simulink model "Proj_10"  (R2017a)
settings: Solver=ode4  StartTime=0.0  StopTime=1000  FixedStep=1  RelTol=1e-3  EnableMultiTasking=on
undefined symbols (not defined in the file or in its folder): ess, mc
libraries: simulink x1
settings Model: Creator=chok1124  LastModifiedBy=Jinesh
settings OptimizationCC: LifeSpan=inf
settings DebuggingCC: SFUnexpectedBacktrackingDiag=warning  SFNoUnconditionalDefaultTransitionDiag=warning  SFExecutionAtInitializationDiag=none
settings GRTTargetCC: TargetLangStandard=C89/C90 (ANSI)  GeneratePreprocessorConditionals=Disable all
settings ConfigComp: CovMetricSettings=dw  CovHtmlReporting=on  CovSaveCumulativeToWorkspaceVar=on  CovSaveSingleToWorkspaceVar=on  CovExternalEMLEnable=off

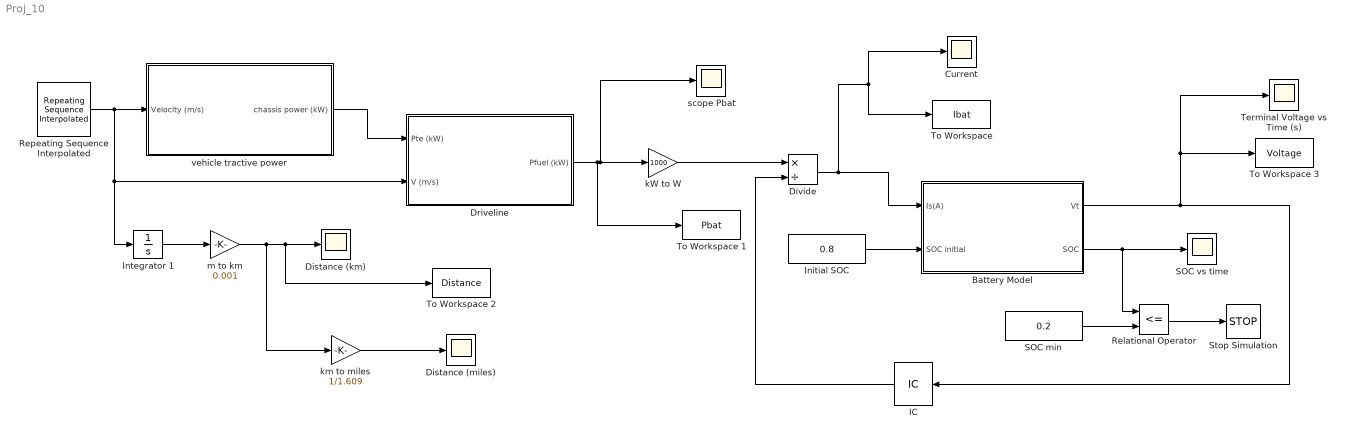
== system Proj_10 ==
  Battery Model : Subsystem
  Current : Scope
  Distance (km) : Scope
  Distance (miles) : Scope
  Divide : Product  Inputs=*/
  Driveline : Subsystem
  IC : InitialCondition  Value=345
  Initial SOC : Constant  Value=0.8
  Integrator 1 : Integrator
  Relational Operator : RelationalOperator  Operator=<=  OutDataTypeStr=boolean  RndMeth=Nearest
  Repeating Sequence Interpolated : simulink/Sources/Repeating Sequence Interpolated  OutValues=V  TimeValues=t  LookUpMeth=Interpolation-Use End Values  tsamp=1  OutMin=[]  OutMax=[]  OutDataTypeStr=double  OutputDataTypeScalingMode=double  OutDataType=fixdt(0,8)  OutScaling=2^-10
  SOC min : Constant  Value=0.2
  SOC vs time : Scope
  Stop Simulation : Stop
  Terminal Voltage vs Time (s) : Scope
  To Workspace : ToWorkspace  VariableName=Ibat  SaveFormat=Timeseries  SampleTime=-1
  To Workspace 1 : ToWorkspace  VariableName=Pbat  SaveFormat=Timeseries  SampleTime=-1
  To Workspace 2 : ToWorkspace  VariableName=Distance  SaveFormat=Timeseries  SampleTime=-1
  To Workspace 3 : ToWorkspace  VariableName=Voltage  SaveFormat=Timeseries  SampleTime=-1
  kW to W : Gain  Gain=1000
  km to miles : Gain  Gain=1/1.609
  m to km : Gain  Gain=0.001
  scope Pbat : Scope
  vehicle tractive power : Subsystem
  wires:
  Divide/1 -> Battery Model/1(Is(A)), To Workspace/1, Current/1
  Initial SOC/1 -> Battery Model/2(SOC initial)
  Battery Model/1(Vt) -> To Workspace 3/1, Terminal Voltage vs Time (s)/1, IC/1
  Battery Model/2(SOC) -> Relational Operator/1, SOC vs time/1
  SOC min/1 -> Relational Operator/2
  Relational Operator/1 -> Stop Simulation/1
  Repeating Sequence Interpolated/1 -> vehicle tractive power/1(Velocity (m/s)), Integrator 1/1, Driveline/2(V (m/s))
  Integrator 1/1 -> m to km/1
  m to km/1 -> Distance (km)/1, To Workspace 2/1, km to miles/1
  vehicle tractive power/1(chassis power (kW)) -> Driveline/1(Pte (kW))
  Driveline/1(Pfuel (kW)) -> kW to W/1, scope Pbat/1, To Workspace 1/1
  km to miles/1 -> Distance (miles)/1
  kW to W/1 -> Divide/1
  IC/1 -> Divide/2

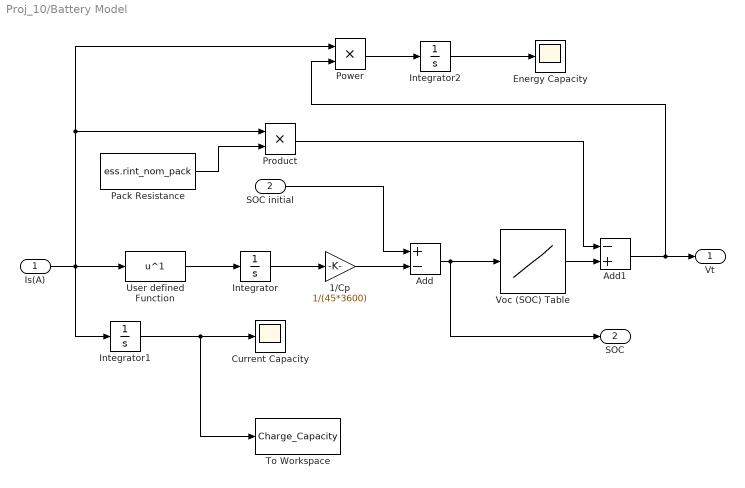
== system Proj_10/Battery Model ==
  Is(A) : Inport
  SOC initial : Inport  Port=2
  1/Cp : Gain  Gain=1/(45*3600)
  Add : Sum  Inputs=+-
  Add1 : Sum  Inputs=-+
  Current Capacity : Scope
  Energy Capacity : Scope
  Integrator : Integrator
  Integrator1 : Integrator
  Integrator2 : Integrator
  Pack Resistance : Constant  Value=ess.rint_nom_pack
  Power : Product
  Product : Product
  To Workspace : ToWorkspace  VariableName=Charge_Capacity  SaveFormat=Timeseries  SampleTime=-1
  User defined Function : Fcn  Expr=u^1
  Voc (SOC) Table : Lookup_n-D  NumberOfTableDimensions=1  BreakpointsForDimension1=ess.soc_index  Table=ess.voc_map_pack  InternalRulePriority=Speed  RndMeth=Simplest  InputSameDT=on
  Vt : Outport
  SOC : Outport  Port=2
  wires:
  Integrator/1 -> 1/Cp/1
  Is(A)/1 -> Integrator1/1, User defined Function/1, Power/1, Product/1
  User defined Function/1 -> Integrator/1
  1/Cp/1 -> Add/2
  SOC initial/1 -> Add/1
  Pack Resistance/1 -> Product/2
  Product/1 -> Add1/1
  Add/1 -> SOC/1, Voc (SOC) Table/1
  Add1/1 -> Power/2, Vt/1
  Voc (SOC) Table/1 -> Add1/2
  Integrator1/1 -> To Workspace/1, Current Capacity/1
  Power/1 -> Integrator2/1
  Integrator2/1 -> Energy Capacity/1

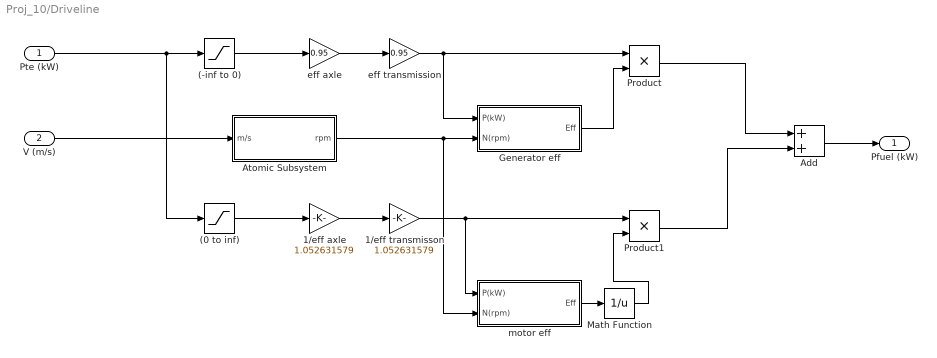
== system Proj_10/Driveline ==
  Pte (kW) : Inport
  V (m/s) : Inport  Port=2
  (-inf to 0) : Saturate  UpperLimit=0  LowerLimit=-inf
  (0 to inf) : Saturate  UpperLimit=inf  LowerLimit=0
  "1/eff axle " : Gain  Gain=1.052631579
  1/eff transmisson : Gain  Gain=1.052631579
  Add : Sum
  Atomic Subsystem : Subsystem  TreatAsAtomicUnit=on
  Generator eff : Subsystem  TreatAsAtomicUnit=on
  Math Function : Math  Operator=reciprocal  SaturateOnIntegerOverflow=on
  Product : Product
  Product1 : Product
  eff axle : Gain  Gain=0.95
  eff transmission : Gain  Gain=0.95
  motor eff : Subsystem  TreatAsAtomicUnit=on
  Pfuel (kW) : Outport
  wires:
  Add/1 -> Pfuel (kW)/1
  V (m/s)/1 -> Atomic Subsystem/1(m/s)
  Pte (kW)/1 -> (0 to inf)/1, (-inf to 0)/1
  eff axle/1 -> eff transmission/1
  "1/eff axle "/1 -> 1/eff transmisson/1
  (-inf to 0)/1 -> eff axle/1
  (0 to inf)/1 -> "1/eff axle "/1
  Atomic Subsystem/1(rpm) -> motor eff/2(N(rpm)), Generator eff/2(N(rpm))
  eff transmission/1 -> Product/1, Generator eff/1(P(kW))
  1/eff transmisson/1 -> motor eff/1(P(kW)), Product1/1
  Generator eff/1("Eff ") -> Product/2
  motor eff/1("Eff ") -> Math Function/1
  Math Function/1 -> Product1/2
  Product/1 -> Add/1
  Product1/1 -> Add/2

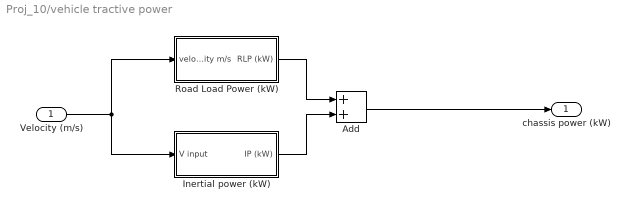
== system Proj_10/vehicle tractive power ==
  Velocity (m/s) : Inport
  Add : Sum
  Inertial power (kW) : Subsystem  TreatAsAtomicUnit=on
  Road Load Power (kW) : Subsystem  TreatAsAtomicUnit=on
  chassis power (kW) : Outport
  wires:
  Velocity (m/s)/1 -> Road Load Power (kW)/1("velocity m/s "), Inertial power (kW)/1(V input)
  Inertial power (kW)/1(IP (kW)) -> Add/2
  Road Load Power (kW)/1(RLP (kW)) -> Add/1
  Add/1 -> chassis power (kW)/1

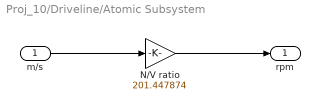
== system Proj_10/Driveline/Atomic Subsystem ==
  m/s : Inport
  N/V ratio : Gain  Gain=201.447874
  rpm : Outport
  wires:
  m/s/1 -> N/V ratio/1
  N/V ratio/1 -> rpm/1

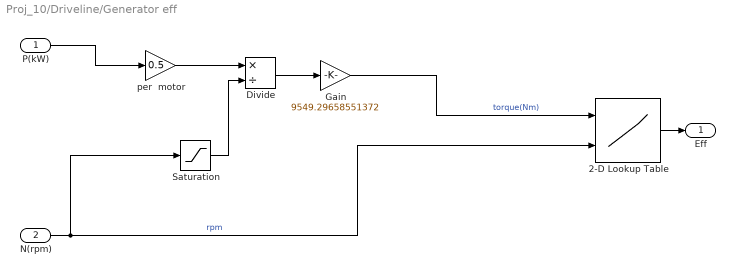
== system Proj_10/Driveline/Generator eff ==
  P(kW) : Inport
  N(rpm) : Inport  Port=2
  2-D Lookup Table : Lookup_n-D  BreakpointsForDimension1=mc.trq_eff_index_gen  BreakpointsForDimension2=mc.rpm_eff_index_gen  Table=mc.eff_trq_map_gen'  InternalRulePriority=Speed  RndMeth=Simplest  InputSameDT=on
  Divide : Product  Inputs=*/
  Gain : Gain  Gain=9549.29658551372
  Saturation : Saturate  UpperLimit=8000  LowerLimit=0.1
  per  motor : Gain  Gain=0.5
  "Eff " : Outport
  wires:
  P(kW)/1 -> per  motor/1
  Divide/1 -> Gain/1
  2-D Lookup Table/1 -> "Eff "/1
  N(rpm)/1 -> 2-D Lookup Table/2, Saturation/1  "rpm"
  Saturation/1 -> Divide/2
  Gain/1 -> 2-D Lookup Table/1  "torque(Nm)"
  per  motor/1 -> Divide/1

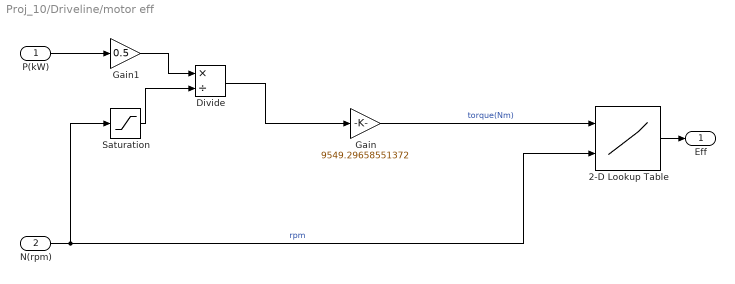
== system Proj_10/Driveline/motor eff ==
  P(kW) : Inport
  N(rpm) : Inport  Port=2
  2-D Lookup Table : Lookup_n-D  BreakpointsForDimension1=mc.trq_eff_index  BreakpointsForDimension2=mc.rpm_eff_index  Table=mc.eff_trq_map'  InternalRulePriority=Speed  RndMeth=Simplest  InputSameDT=on
  Divide : Product  Inputs=*/
  Gain : Gain  Gain=9549.29658551372
  Gain1 : Gain  Gain=0.5
  Saturation : Saturate  UpperLimit=8000  LowerLimit=0.1
  "Eff " : Outport
  wires:
  P(kW)/1 -> Gain1/1
  Divide/1 -> Gain/1
  2-D Lookup Table/1 -> "Eff "/1
  Gain/1 -> 2-D Lookup Table/1  "torque(Nm)"
  N(rpm)/1 -> Saturation/1, 2-D Lookup Table/2  "rpm"
  Saturation/1 -> Divide/2
  Gain1/1 -> Divide/1

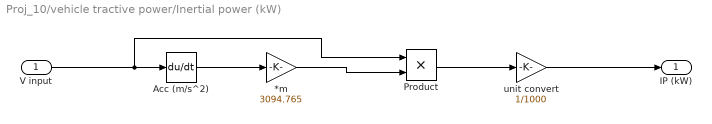
== system Proj_10/vehicle tractive power/Inertial power (kW) ==
  V input : Inport
  *m : Gain  Gain=3094.765
  Acc (m/s^2) : Derivative
  Product : Product
  unit convert : Gain  Gain=1/1000
  IP (kW) : Outport
  wires:
  V input/1 -> Product/1, Acc (m/s^2)/1
  Acc (m/s^2)/1 -> *m/1
  *m/1 -> Product/2
  Product/1 -> unit convert/1
  unit convert/1 -> IP (kW)/1

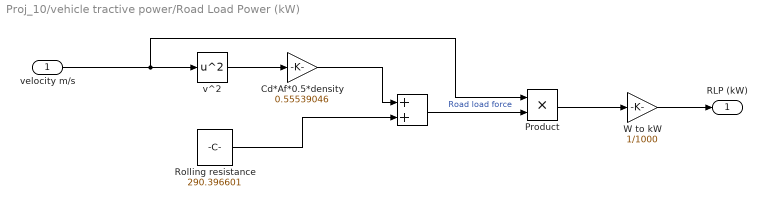
== system Proj_10/vehicle tractive power/Road Load Power (kW) ==
  "velocity m/s " : Inport
  " " : Sum
  "Cd*Af*0.5*density " : Gain  Gain=0.55539046
  Product : Product
  "Rolling resistance " : Constant  Value=290.396601
  W to kW : Gain  Gain=1/1000
  v^2 : Math  Operator=square  SaturateOnIntegerOverflow=on
  RLP (kW) : Outport
  wires:
  v^2/1 -> "Cd*Af*0.5*density "/1
  "velocity m/s "/1 -> Product/1, v^2/1
  "Cd*Af*0.5*density "/1 -> " "/1
  "Rolling resistance "/1 -> " "/2
  " "/1 -> Product/2  "Road load force"
  Product/1 -> W to kW/1
  W to kW/1 -> RLP (kW)/1
